simulink model "e04_MtrCtrl_PwmSet"  (R2024a)
settings: Solver=FixedStepDiscrete  StartTime=0.0  StopTime=1  FixedStep=mSim.dTime  MaxStep=Define.sModelSampleTime  RelTol=7.1420e-05
undefined symbols (not defined in the file): Cnst, CnstCnst, E04VTDC
libraries: Lib_LPF x1
settings Model: Creator=user  LastModifiedBy=admin
settings SolverCC: MaxConsecutiveZCs=10000  ZeroCrossAlgorithm=Adaptive  AlgebraicLoopSolver=TrustRegion
settings DataIOCC: SaveOutput=off  DSMLogging=off  InspectSignalLogs=on  SaveTime=off  SignalLoggingName=logsout_Validator
settings OptimizationCC: BlockReduction=off  DefaultParameterBehavior=Inlined  UseDivisionForNetSlopeComputation=UseDivisionForReciprocalsOfIntegersOnly  GainParamInheritBuiltInType=on  UseFloatMulNetSlope=on  DefaultUnderspecifiedDataType=single  InlineInvariantSignals=on  BitwiseOrLogicalOp=Logical operator  PassReuseOutputArgsAs=Individual arguments  EfficientFloat2IntCast=on  LifeSpan=Inf  OptimizeBlockOrder=speed  DifferentSizesBufferReuse=on  EfficientTunableParamExpr=on
settings DebuggingCC: SignalInfNanChecking=error  SignalRangeChecking=error  ReadBeforeWriteMsg=EnableAllAsError  WriteAfterWriteMsg=EnableAllAsError  WriteAfterReadMsg=EnableAllAsError  AlgebraicLoopMsg=error  ArtificialAlgebraicLoopMsg=error  SaveWithDisabledLinksMsg=error  SaveWithParameterizedLinksMsg=error  BlockPriorityViolationMsg=error  SolverPrmCheckMsg=error  InheritedTsInSrcMsg=error  SingleTaskRateTransMsg=error  TasksWithSamePriorityMsg=error  SigSpecEnsureSampleTimeMsg=error  CheckMatrixSingularityMsg=error  IntegerOverflowMsg=error  ParameterUnderflowMsg=error  ParameterPrecisionLossMsg=error  ParameterTunabilityLossMsg=error  UnderSpecifiedDataTypeMsg=error  UnnecessaryDatatypeConvMsg=warning  VectorMatrixConversionMsg=error  SignalLabelMismatchMsg=error  UnconnectedInputMsg=error  UnconnectedOutputMsg=error  UnconnectedLineMsg=error  SFcnCompatibilityMsg=error  UniqueDataStoreMsg=error  BusObjectLabelMismatch=error  RootOutportRequireBusObject=error  AssertControl=DisableAll  ModelReferenceIOMismatchMessage=error  UnknownTsInhSupMsg=error  ModelReferenceDataLoggingMessage=error  ModelReferenceSymbolNameMessage=none  StateNameClashWarn=warning  StrictBusMsg=ErrorOnBusTreatedAsVector  NonBusSignalsTreatedAsBus=error  SFInvalidInputDataAccessInChartInitDiag=error  SFTransitionOutsideNaturalParentDiag=error  SFUnreachableExecutionPathDiag=error  SFUndirectedBroadcastEventsDiag=error  SFTransitionActionBeforeConditionDiag=error  SFTemporalDelaySmallerThanSampleTimeDiag=error  SFSelfTransitionDiag=error  SFExecutionAtInitializationDiag=error  IntegerSaturationMsg=error  UnitsInconsistencyMsg=none  VariantConditionMismatch=error
settings HardwareCC: ProdBitPerChar=16  ProdBitPerInt=16  ProdBitPerPointer=32  ProdBitPerSizeT=32  ProdBitPerPtrDiffT=32  ProdLargestAtomicInteger=Integer  ProdLargestAtomicFloat=None  ProdWordSize=16  ProdLongLongMode=on  ProdHWDeviceType=Texas Instruments->C2000
settings ModelReferenceCC: EnableRefExpFcnMdlSchedulingChecks=on  ModelReferenceNumInstancesAllowed=Single
settings SFSimCC: SimUseLocalCustomCode=off  CompileTimeRecursionLimit=0  EnableRuntimeRecursion=off  MATLABDynamicMemAlloc=off  CustomCodeUndefinedFunction=UseInterfaceOnly
settings RTWCC: Description=Embedded Coder  SystemTargetFile=ert.tlc  GenCodeOnly=on  TemplateMakefile=ert_default_tmf  GenerateReport=on  RTWUseLocalCustomCode=off  BuildConfiguration=Faster Runs  IncludeHyperlinkInReport=on  LaunchReport=on  GenerateTraceInfo=on  GenerateTraceReport=on  GenerateTraceReportSl=on  GenerateTraceReportSf=on  GenerateWebview=on  GenerateCodeMetricsReport=on  GenerateCodeReplacementReport=on  GPUComputeCapability=3.5  DLArmComputeVersion=19.05
settings CodeAppCC: ForceParamTrailComments=on  IgnoreCustomStorageClasses=off  MATLABFcnDesc=on  MangleLength=4  CustomSymbolStrGlobalVar=GvE04$N$M  CustomSymbolStrType=StrE04$N$M  CustomSymbolStrFcn=$N$M$F  CustomSymbolStrMacro=$N$M  DefineNamingRule=UpperCase  ParamNamingRule=UpperCase  SimulinkBlockComments=off  MATLABSourceComments=on  EnableCustomComments=on  ReqsInCode=on
settings ERTTargetCC: TargetLangStandard=C99 (ISO)  UtilityFuncGeneration=Shared location  MultiwordLength=2048  IncludeMdlTerminateFcn=off  CombineSignalStateStructs=on  SuppressErrorStatus=on  SupportAbsoluteTime=off  SupportNonFinite=off  ParenthesesLevel=Maximum  CastingMode=Standards  GenerateSharedConstants=off  InlinedParameterPlacement=NonHierarchical  ERTSrcFileBannerTemplate=t_code_template.cgt  ERTHdrFileBannerTemplate=t_code_template.cgt  ERTDataSrcFileTemplate=t_code_template.cgt  ERTDataHdrFileTemplate=t_code_template.cgt  ERTCustomFileTemplate=example_file_process.tlc  ERTFilePackagingFormat=CompactWithDataFile  PreserveExpressionOrder=on  SuppressUnreachableDefaultCases=off  EnableSignedLeftShifts=off  EnableSignedRightShifts=off  IndentStyle=Allman  IndentSize=4
settings ConfigComp: CovSaveName=coveragedata  CovMetricSettings=we  CovEnableCumulative=off  CovSaveCumulativeToWorkspaceVar=on  CovSaveSingleToWorkspaceVar=on  CovOutputDir=sldv_output/$ModelName$\sldv_covoutput  PSVerificationMode=BugFinder  PSModelRefIgnoreList=[]  PSEnableModelRefIgnoreList=off  PSModelRefMinMaxVerif=CheckAndConstrain  PSAutoStubLUT=on  DVModelCoverageObjectives=MCDC  DVTestSuiteOptimization=CombinedObjectives (Nonlinear Extended)  DVRebuildModelRepresentation=Always
settings SimscapeCC: SimscapeNormalizeSystem=off

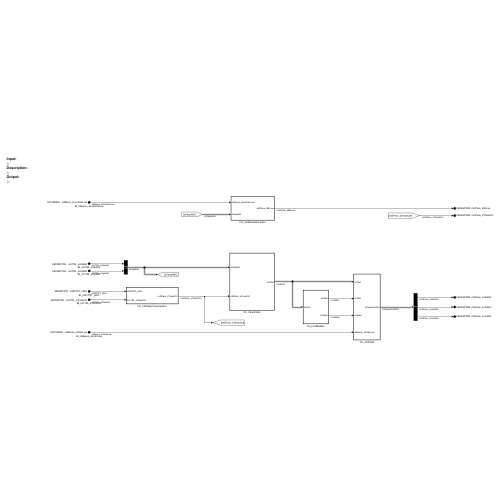
[thumbnail: Simulink's stored preview of the top-level diagram]
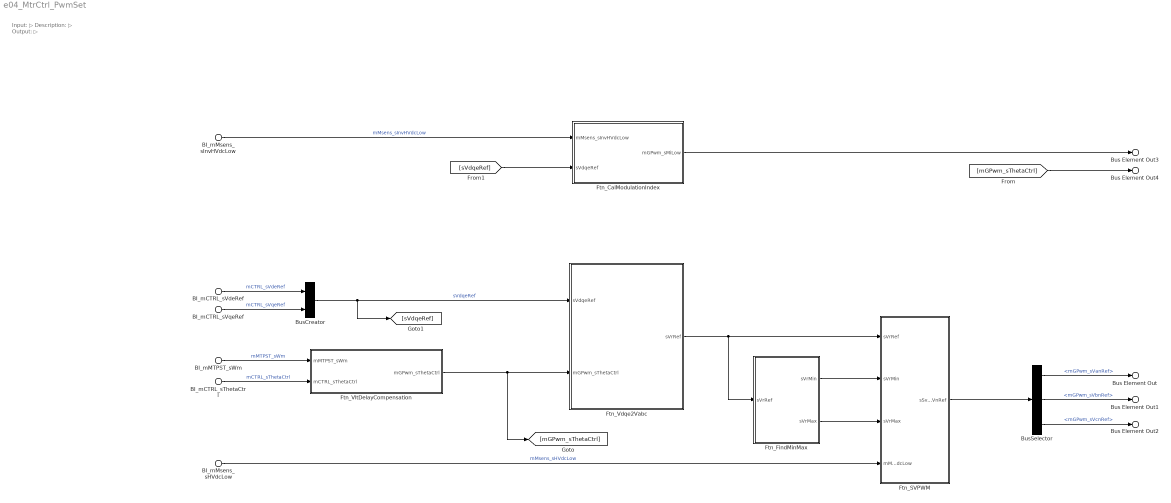
== system e04_MtrCtrl_PwmSet ==
  note: Input:
      | ▷
      | Description:
      | ▷
      | Output:
      | ▷
  BI_mMsens_sHVdcLow : Inport  Description=■ 설명: DC Link 전압  PortName=bC01MADC  Element=mMsens_sHVdcLow
  BI_mMsens_sInvHVdcLow : Inport  Description=■ 설명: DC Link 전압 역수  PortName=bC01MADC  Element=mMsens_sInvHVdcLow
  BI_mMTPST_sWm : Inport  Description=■ 설명: 기계 각속도 (Wm = 12000 * 2pi/60)  Port=2  PortName=bE02MTPST  Element=mMTPST_sWm
  BI_mCTRL_sVdeRef : Inport  Description=■ 설명: Vde Reference  Port=3  PortName=bE03MCTRL  Element=mCTRL_sVdeRef
  BI_mCTRL_sVqeRef : Inport  Description=■ 설명: Vqe Reference  Port=3  PortName=bE03MCTRL  Element=mCTRL_sVqeRef
  BI_mCTRL_sThetaCtrl : Inport  Description=■ 설명: 모터 회전자 위치  Port=3  PortName=bE03MCTRL  Element=mCTRL_sThetaCtrl
  BusCreator : BusCreator  Inputs=2
  BusSelector : BusSelector  OutputSignals=mGPwm_sVanRef,mGPwm_sVbnRef,mGPwm_sVcnRef
  Ftn_CalModulationIndex : Subsystem  TreatAsAtomicUnit=on
      settings: RTWSystemCode=Nonreusable function  RTWFcnNameOpts=Use subsystem name
  Ftn_FindMinMax : Subsystem  TreatAsAtomicUnit=on
      settings: RTWSystemCode=Nonreusable function  RTWFcnNameOpts=Use subsystem name
  Ftn_SVPWM : Subsystem  TreatAsAtomicUnit=on
      settings: RTWSystemCode=Nonreusable function  RTWFcnNameOpts=Use subsystem name
  Ftn_Vdqe2Vabc : Subsystem  TreatAsAtomicUnit=on
      settings: RTWSystemCode=Nonreusable function  RTWFcnNameOpts=Use subsystem name
  Ftn_VltDelayCompensation : Subsystem  TreatAsAtomicUnit=on
      settings: RTWSystemCode=Nonreusable function  RTWFcnNameOpts=Use subsystem name
  Bus Element Out : Outport  Description=■ 설명: A Phase Voltage Reference  PortName=bE04GPWM  Element=mGPwm_sVanRef
  Bus Element Out1 : Outport  Description=■ 설명: B Phase Voltage Reference  PortName=bE04GPWM  Element=mGPwm_sVbnRef
  Bus Element Out2 : Outport  Description=■ 설명: C Phase Voltage Reference  PortName=bE04GPWM  Element=mGPwm_sVcnRef
  Bus Element Out3 : Outport  Description=■ 설명: Modulation Index  PortName=bE04GPWM  Element=mGPwm_sMiLow
  Bus Element Out4 : Outport  Description=■ 설명: Modulation Index  PortName=bE04GPWM  Element=mGPwm_sThetaCtrl
  wires:
  Ftn_CalModulationIndex/1(mGPwm_sMiLow) -> Bus Element Out3/1
  Ftn_FindMinMax/2(sVrMax) -> Ftn_SVPWM/3(sVrMax)
  BI_mCTRL_sVdeRef/1 -> BusCreator/1  "mCTRL_sVdeRef"
  [sVdqeRef] -> Ftn_CalModulationIndex/2(sVdqeRef)
  BI_mMsens_sHVdcLow/1 -> Ftn_SVPWM/4(mMsens_sHVdcLow)  "mMsens_sHVdcLow"
  Ftn_FindMinMax/1(sVrMin) -> Ftn_SVPWM/2(sVrMin)
  BusSelector/2 -> Bus Element Out1/1  "<mGPwm_sVbnRef>"
  [mGPwm_sThetaCtrl] -> Bus Element Out4/1
  BI_mMsens_sInvHVdcLow/1 -> Ftn_CalModulationIndex/1(mMsens_sInvHVdcLow)  "mMsens_sInvHVdcLow"
  BusSelector/1 -> Bus Element Out/1  "<mGPwm_sVanRef>"
  BI_mMTPST_sWm/1 -> Ftn_VltDelayCompensation/1(mMTPST_sWm)  "mMTPST_sWm"
  BusCreator/1 -> [sVdqeRef], Ftn_Vdqe2Vabc/1(sVdqeRef)  "sVdqeRef"
  BusSelector/3 -> Bus Element Out2/1  "<mGPwm_sVcnRef>"
  Ftn_VltDelayCompensation/1(mGPwm_sThetaCtrl) -> [mGPwm_sThetaCtrl], Ftn_Vdqe2Vabc/2(mGPwm_sThetaCtrl)
  BI_mCTRL_sVqeRef/1 -> BusCreator/2  "mCTRL_sVqeRef"
  Ftn_Vdqe2Vabc/1(sVrRef) -> Ftn_SVPWM/1(sVrRef), Ftn_FindMinMax/1(sVrRef)
  Ftn_SVPWM/1(sSvpwmVnRef) -> BusSelector/1
  BI_mCTRL_sThetaCtrl/1 -> Ftn_VltDelayCompensation/2(mCTRL_sThetaCtrl)  "mCTRL_sThetaCtrl"

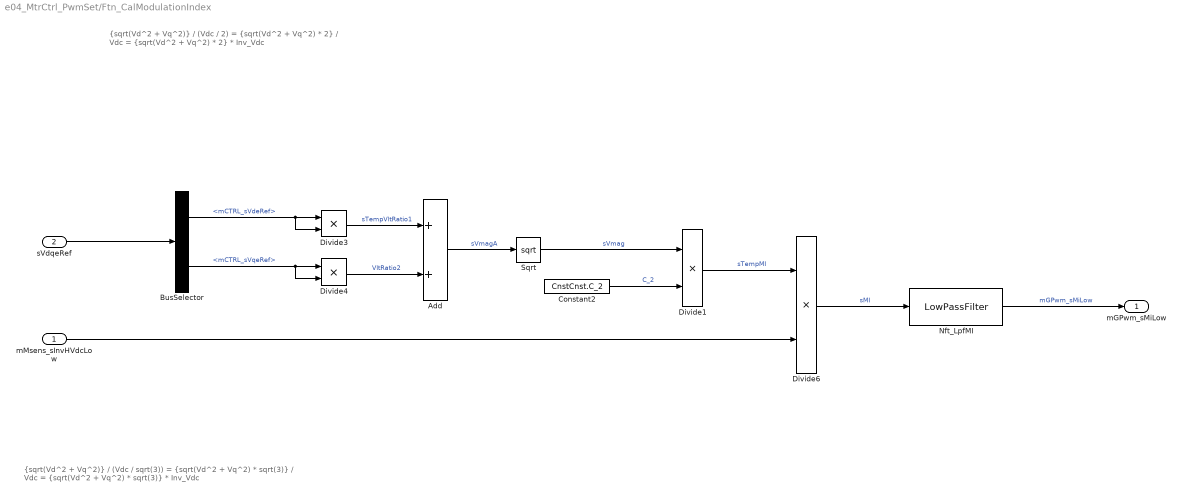
== system e04_MtrCtrl_PwmSet/Ftn_CalModulationIndex ==
  note: {sqrt(Vd^2 + Vq^2)} / (Vdc / sqrt(3))
      | = {sqrt(Vd^2 + Vq^2) * sqrt(3)} / Vdc
      | = {sqrt(Vd^2 + Vq^2) * sqrt(3)} * Inv_Vdc
  note: {sqrt(Vd^2 + Vq^2)} / (Vdc / 2)
      | = {sqrt(Vd^2 + Vq^2) * 2} / Vdc
      | = {sqrt(Vd^2 + Vq^2) * 2} * Inv_Vdc
  mMsens_sInvHVdcLow : Inport
  sVdqeRef : Inport  Port=2
  Add : Sum
  BusSelector : BusSelector  OutputSignals=mCTRL_sVdeRef,mCTRL_sVqeRef
  Constant2 : Constant  Value=CnstCnst.C_2  OutDataTypeStr=single
  Divide{1,3..4,6} (4 alike) : Product  Inputs=**
  Nft_LpfMI : Lib_LPF/LowPassFilter  La=E04SWF.sVltRatioLa  Lb=E04SWF.sVltRatioLb  Init_Value=0
  Sqrt : Sqrt
  mGPwm_sMiLow : Outport
  wires:
  sVdqeRef/1 -> BusSelector/1
  BusSelector/1 -> Divide3/2, Divide3/1  "<mCTRL_sVdeRef>"
  BusSelector/2 -> Divide4/2, Divide4/1  "<mCTRL_sVqeRef>"
  Divide3/1 -> Add/1  "sTempVltRatio1"
  Divide4/1 -> Add/2  "VltRatio2"
  Add/1 -> Sqrt/1  "sVmagA"
  Divide1/1 -> Divide6/1  "sTempMI"
  mMsens_sInvHVdcLow/1 -> Divide6/2
  Constant2/1 -> Divide1/2  "C_2"
  Divide6/1 -> Nft_LpfMI/1  "sMI"
  Sqrt/1 -> Divide1/1  "sVmag"
  Nft_LpfMI/1 -> mGPwm_sMiLow/1  "mGPwm_sMiLow"

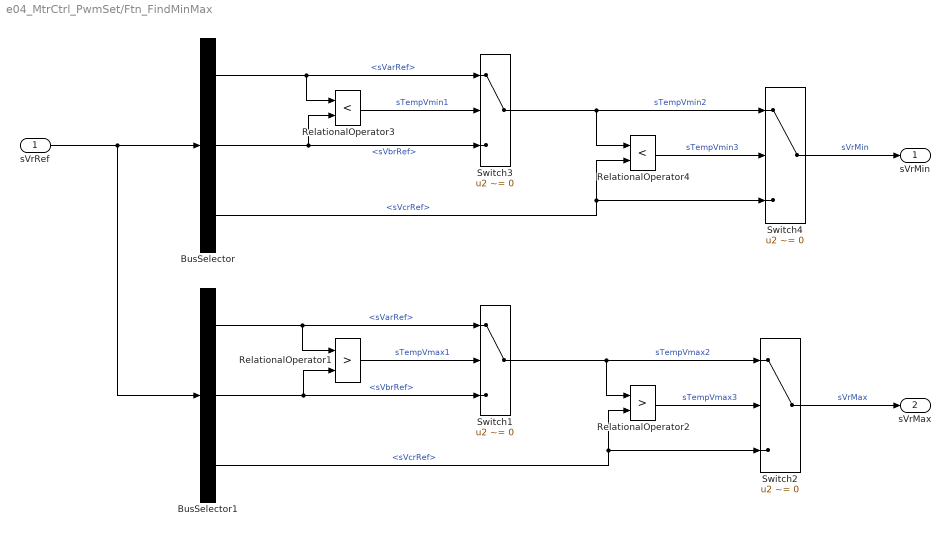
== system e04_MtrCtrl_PwmSet/Ftn_FindMinMax ==
  sVrRef : Inport
  BusSelector : BusSelector  OutputSignals=sVarRef,sVbrRef,sVcrRef
  BusSelector1 : BusSelector  OutputSignals=sVarRef,sVbrRef,sVcrRef
  RelationalOperator1 : RelationalOperator  Operator=>  InputSameDT=off
  RelationalOperator2 : RelationalOperator  Operator=>  InputSameDT=off
  RelationalOperator3 : RelationalOperator  Operator=<  InputSameDT=off
  RelationalOperator4 : RelationalOperator  Operator=<  InputSameDT=off
  Switch{1..4} (4 alike) : Switch  Criteria=u2 ~= 0  SaturateOnIntegerOverflow=off  InputSameDT=off
  sVrMin : Outport  VectorParamsAs1DForOutWhenUnconnected=off
  sVrMax : Outport  Port=2  VectorParamsAs1DForOutWhenUnconnected=off
  wires:
  RelationalOperator4/1 -> Switch4/2  "sTempVmin3"
  RelationalOperator3/1 -> Switch3/2  "sTempVmin1"
  Switch3/1 -> RelationalOperator4/1, Switch4/1  "sTempVmin2"
  sVrRef/1 -> BusSelector1/1, BusSelector/1
  BusSelector/1 -> Switch3/1, RelationalOperator3/1  "<sVarRef>"
  BusSelector/3 -> RelationalOperator4/2, Switch4/3  "<sVcrRef>"
  BusSelector/2 -> Switch3/3, RelationalOperator3/2  "<sVbrRef>"
  Switch4/1 -> sVrMin/1  "sVrMin"
  Switch2/1 -> sVrMax/1  "sVrMax"
  Switch1/1 -> RelationalOperator2/1, Switch2/1  "sTempVmax2"
  BusSelector1/2 -> RelationalOperator1/2, Switch1/3  "<sVbrRef>"
  RelationalOperator1/1 -> Switch1/2  "sTempVmax1"
  RelationalOperator2/1 -> Switch2/2  "sTempVmax3"
  BusSelector1/1 -> RelationalOperator1/1, Switch1/1  "<sVarRef>"
  BusSelector1/3 -> RelationalOperator2/2, Switch2/3  "<sVcrRef>"

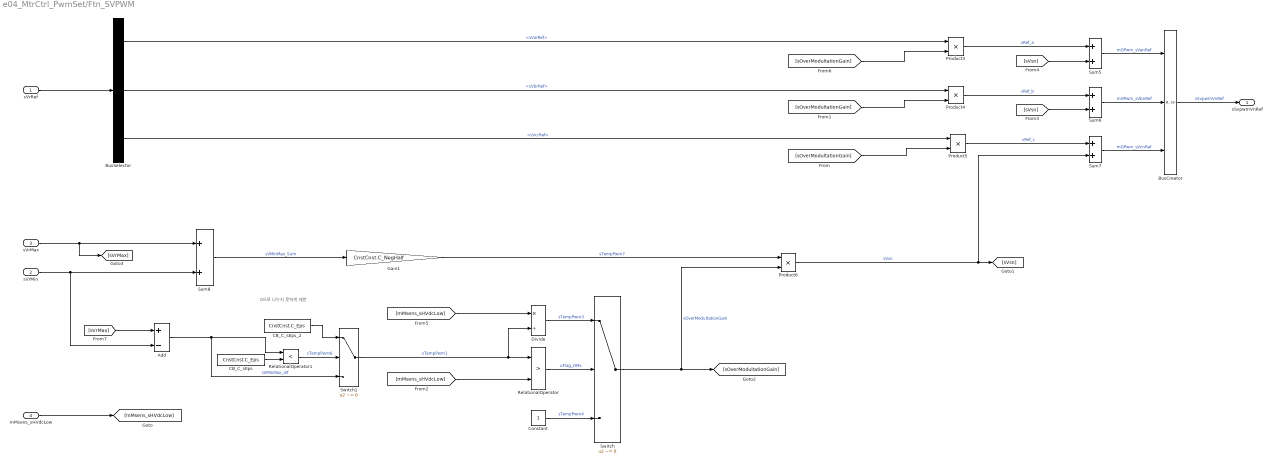
== system e04_MtrCtrl_PwmSet/Ftn_SVPWM ==
  note: 0으로 나누지 못하게 제한
  sVrRef : Inport
  sVrMin : Inport  Port=2
  sVrMax : Inport  Port=3
  mMsens_sHVdcLow : Inport  Port=4
  Add : Sum  Inputs=+-
  BusCreator : BusCreator  Inputs=3
  BusSelector : BusSelector  OutputSignals=sVarRef,sVbrRef,sVcrRef
  CB_C_sEps : Constant  Value=CnstCnst.C_Eps
  CB_C_sEps_2 : Constant  Value=CnstCnst.C_Eps
  Constant : Constant  OutDataTypeStr=single
  Divide : Product  Inputs=*/
  Gain1 : Gain  Gain=CnstCnst.C_NegHalf  ParamDataTypeStr=single
  Product{3..6} (4 alike) : Product  RndMeth=Zero
  RelationalOperator : RelationalOperator  Operator=>  InputSameDT=off
  RelationalOperator1 : RelationalOperator  Operator=<  RndMeth=Floor  InputSameDT=off
  Sum{5..8} (4 alike) : Sum
  Switch : Switch  Criteria=u2 ~= 0  SaturateOnIntegerOverflow=off  InputSameDT=off
  Switch1 : Switch  Criteria=u2 ~= 0  SaturateOnIntegerOverflow=off  InputSameDT=off
  sSvpwmVnRef : Outport
  wires:
  Sum7/1 -> BusCreator/3  "mGPwm_sVcnRef"
  Sum6/1 -> BusCreator/2  "mGPwm_sVbnRef"
  Sum5/1 -> BusCreator/1  "mGPwm_sVanRef"
  BusCreator/1 -> sSvpwmVnRef/1  "sSvpwmVnRef"
  sVrRef/1 -> BusSelector/1
  Divide/1 -> Switch/1  "sTempPwm3"
  Product3/1 -> Sum5/1  "vRef_a"
  Add/1 -> RelationalOperator1/1, Switch1/3  "sVMinMax_dif"
  sVrMax/1 -> [sVrMax], Sum8/1
  Product5/1 -> Sum7/1  "vRef_c"
  RelationalOperator/1 -> Switch/2  "uFlag_OMx"
  [mMsens_sHVdcLow] -> RelationalOperator/2
  Switch/1 -> [sOverModultationGain], Product6/2  "sOverModultationGain"
  BusSelector/1 -> Product3/1  "<sVarRef>"
  BusSelector/3 -> Product5/1  "<sVcrRef>"
  BusSelector/2 -> Product4/1  "<sVbrRef>"
  Sum8/1 -> Gain1/1  "sVMinMax_Sum"
  Constant/1 -> Switch/3  "sTempPwm4"
  RelationalOperator1/1 -> Switch1/2  "sTempPwm6"
  Product4/1 -> Sum6/1  "vRef_b"
  Switch1/1 -> Divide/2, RelationalOperator/1  "sTempPwm1"
  Product6/1 -> [sVsn], Sum7/2  "sVsn"
  [sVsn] -> Sum5/2
  [sVsn] -> Sum6/2
  mMsens_sHVdcLow/1 -> [mMsens_sHVdcLow]
  [mMsens_sHVdcLow] -> Divide/1
  [sOverModultationGain] -> Product5/2
  [sOverModultationGain] -> Product4/2
  [sOverModultationGain] -> Product3/2
  Gain1/1 -> Product6/1  "sTempPwm7"
  [sVrMax] -> Add/1
  sVrMin/1 -> Add/2, Sum8/2
  CB_C_sEps/1 -> RelationalOperator1/2
  CB_C_sEps_2/1 -> Switch1/1

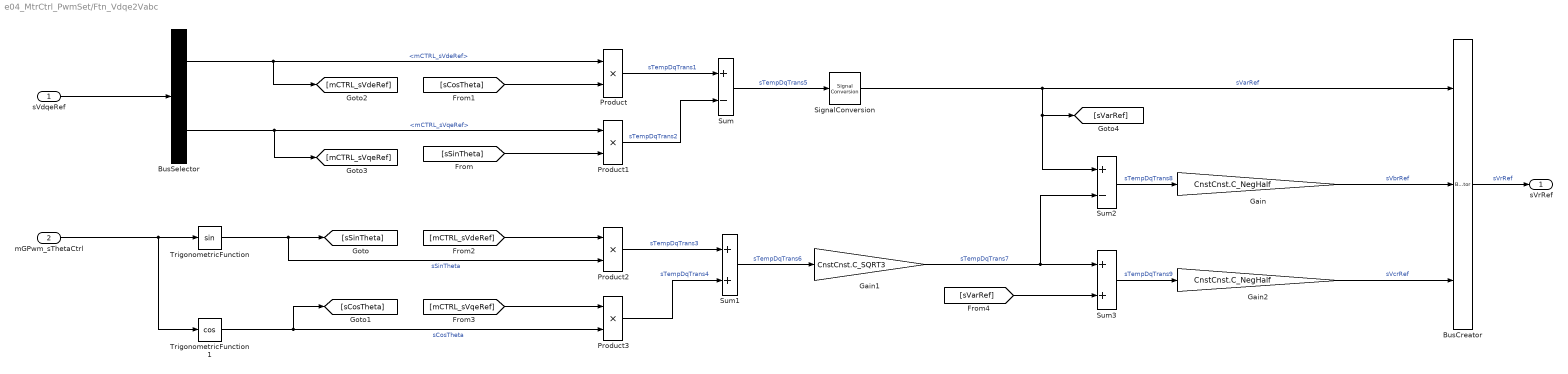
== system e04_MtrCtrl_PwmSet/Ftn_Vdqe2Vabc ==
  sVdqeRef : Inport
  mGPwm_sThetaCtrl : Inport  Port=2
  BusCreator : BusCreator  Inputs=3
  BusSelector : BusSelector  OutputSignals=mCTRL_sVdeRef,mCTRL_sVqeRef
  Gain : Gain  Gain=CnstCnst.C_NegHalf
  Gain1 : Gain  Gain=CnstCnst.C_SQRT3
  Gain2 : Gain  Gain=CnstCnst.C_NegHalf
  Product{,1..3} (4 alike) : Product  RndMeth=Zero
  SignalConversion : SignalConversion  OverrideOpt=off
  Sum : Sum  Inputs=+-
  Sum1 : Sum
  Sum2 : Sum  Inputs=+-
  Sum3 : Sum
  TrigonometricFunction : Trigonometry
  TrigonometricFunction1 : Trigonometry  Operator=cos
  sVrRef : Outport  VectorParamsAs1DForOutWhenUnconnected=off
  wires:
  [mCTRL_sVqeRef] -> Product3/1
  Product1/1 -> Sum/2  "sTempDqTrans2"
  Product3/1 -> Sum1/2  "sTempDqTrans4"
  [sSinTheta] -> Product1/2
  [sCosTheta] -> Product/2
  Sum1/1 -> Gain1/1  "sTempDqTrans6"
  BusCreator/1 -> sVrRef/1  "sVrRef"
  BusSelector/1 -> Product/1, [mCTRL_sVdeRef]  "<mCTRL_sVdeRef>"
  Gain2/1 -> BusCreator/3  "sVcrRef"
  Product2/1 -> Sum1/1  "sTempDqTrans3"
  sVdqeRef/1 -> BusSelector/1
  Gain1/1 -> Sum3/1, Sum2/2  "sTempDqTrans7"
  SignalConversion/1 -> BusCreator/1, [sVarRef], Sum2/1  "sVarRef"
  Product/1 -> Sum/1  "sTempDqTrans1"
  Sum3/1 -> Gain2/1  "sTempDqTrans9"
  Sum2/1 -> Gain/1  "sTempDqTrans8"
  Gain/1 -> BusCreator/2  "sVbrRef"
  Sum/1 -> SignalConversion/1  "sTempDqTrans5"
  mGPwm_sThetaCtrl/1 -> TrigonometricFunction/1, TrigonometricFunction1/1
  TrigonometricFunction/1 -> [sSinTheta], Product2/2  "sSinTheta"
  TrigonometricFunction1/1 -> Product3/2, [sCosTheta]  "sCosTheta"
  [mCTRL_sVdeRef] -> Product2/1
  BusSelector/2 -> [mCTRL_sVqeRef], Product1/1  "<mCTRL_sVqeRef>"
  [sVarRef] -> Sum3/2

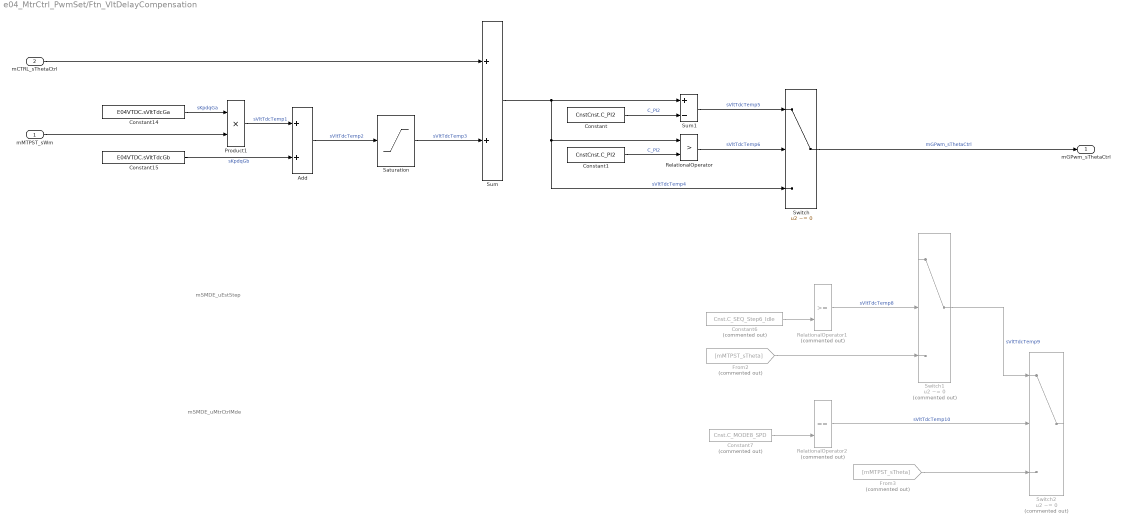
== system e04_MtrCtrl_PwmSet/Ftn_VltDelayCompensation ==
  note: mSMDE_uMtrCtrlMde
  note: mSMDE_uEstStep
  mMTPST_sWm : Inport
  mCTRL_sThetaCtrl : Inport  Port=2
  Add : Sum
  Constant : Constant  Value=CnstCnst.C_PI2
  Constant1 : Constant  Value=CnstCnst.C_PI2
  Constant14 : Constant  Value=E04VTDC.sVltTdcGa
  Constant15 : Constant  Value=E04VTDC.sVltTdcGb
  Constant6 : Constant  Commented=on  Value=Cnst.C_SEQ_Step6_Idle
  Constant7 : Constant  Commented=on  Value=Cnst.C_MODE8_SPD
  From2 : From  Commented=on  GotoTag=mMTPST_sTheta
  From3 : From  Commented=on  GotoTag=mMTPST_sTheta
  Product1 : Product
  RelationalOperator : RelationalOperator  Operator=>  InputSameDT=off
  RelationalOperator1 : RelationalOperator  Commented=on  InputSameDT=off
  RelationalOperator2 : RelationalOperator  Commented=on  Operator===  InputSameDT=off
  Saturation : Saturate  UpperLimit=E04VTDC.sVltTdcRadMax  LowerLimit=E04VTDC.sVltTdcRadMin
      settings: AttributesFormatString=|
      | %<LowerLimit>
      | %<UpperLimit>
  Sum : Sum
  Sum1 : Sum  Inputs=+-
  Switch : Switch  Criteria=u2 ~= 0  SaturateOnIntegerOverflow=off  InputSameDT=off
  Switch1 : Switch  Commented=on  Criteria=u2 ~= 0  SaturateOnIntegerOverflow=off  InputSameDT=off
  Switch2 : Switch  Commented=on  Criteria=u2 ~= 0  SaturateOnIntegerOverflow=off  InputSameDT=off
  mGPwm_sThetaCtrl : Outport
  wires:
  RelationalOperator2/1 -> Switch2/2  "sVltTdcTemp10"
  Constant7/1 -> RelationalOperator2/2
  ? -> RelationalOperator2/1
  Switch1/1 -> Switch2/1  "sVltTdcTemp9"
  mMTPST_sWm/1 -> Product1/2
  ? -> RelationalOperator1/1
  RelationalOperator1/1 -> Switch1/2  "sVltTdcTemp8"
  Constant6/1 -> RelationalOperator1/2
  mCTRL_sThetaCtrl/1 -> Sum/1
  Sum1/1 -> Switch/1  "sVltTdcTemp5"
  Constant/1 -> Sum1/2  "C_PI2"
  Sum/1 -> Switch/3, RelationalOperator/1, Sum1/1  "sVltTdcTemp4"
  RelationalOperator/1 -> Switch/2  "sVltTdcTemp6"
  Switch/1 -> mGPwm_sThetaCtrl/1  "mGPwm_sThetaCtrl"
  From3/1 -> Switch2/3
  From2/1 -> Switch1/3
  Saturation/1 -> Sum/2  "sVltTdcTemp3"
  Product1/1 -> Add/1  "sVltTdcTemp1"
  Constant15/1 -> Add/2  "sKpdqGb"
  Constant14/1 -> Product1/1  "sKpdqGa"
  Add/1 -> Saturation/1  "sVltTdcTemp2"
  Constant1/1 -> RelationalOperator/2  "C_PI2"
